simulink model "tesy"
settings: Solver=VariableStepAuto  StartTime=0.0  StopTime=10.0  RelTol=1e-3
settings SFSimCC: SimCustomHeaderCode="#include \"Main.h\""  SimUserSources=Main.c const.c val.c myAdd.c mySub.c  SimUserIncludeDirs=./src
settings RTWCC: DLArmComputeVersion=19.05

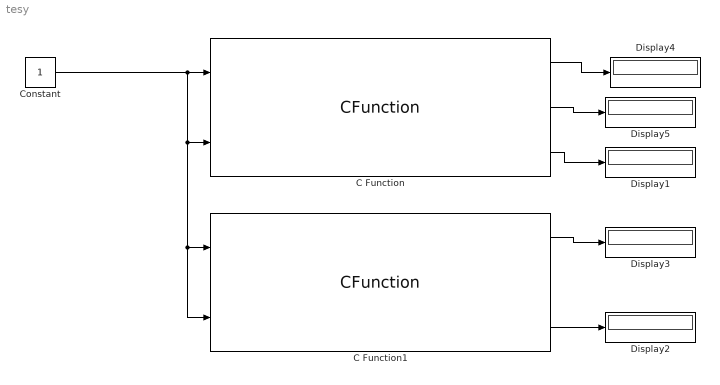
== system tesy ==
  C Function : CFunction  OutputCode=Main2(u1, u2, &y1, &y2, &y3);
  C Function1 : CFunction  OutputCode=Main1(u1, u2, &y1, &y2, &y3);
  Constant : Constant
  Display{1..5} (5 alike) : Display
  wires:
  C Function/1 -> Display4/1
  C Function/2 -> Display5/1
  C Function/3 -> Display1/1
  Constant/1 -> C Function1/2, C Function1/1, C Function/2, C Function/1
  C Function1/3 -> Display2/1
  C Function1/1 -> Display3/1
